simulink model "TEP_Final_NoScript"  (R2024a)
settings: Solver=FixedStepAuto  StartTime=0.0  StopTime=10  FixedStep=1/3600  RelTol=1e-3
model workspace (MAT data in the model file):
  AD : Simulink.Parameter (value not decoded)
  AG : Simulink.Parameter (value not decoded)
  AH : Simulink.Parameter (value not decoded)
  AV : Simulink.Parameter (value not decoded)
  AVP : Simulink.Parameter (value not decoded)
  BCHL : Simulink.Parameter (value not decoded)
  BCHV : Simulink.Parameter (value not decoded)
  BD : Simulink.Parameter (value not decoded)
  BG : Simulink.Parameter (value not decoded)
  BH : Simulink.Parameter (value not decoded)
  BVP : Simulink.Parameter (value not decoded)
  CD : Simulink.Parameter (value not decoded)
  CG : Simulink.Parameter (value not decoded)
  CH : Simulink.Parameter (value not decoded)
  CVP : Simulink.Parameter (value not decoded)
  XMW : Simulink.Parameter (value not decoded)
  XNS : Simulink.Parameter (value not decoded)
  XNSE : Simulink.Parameter (value not decoded)
symbols that are objects in the model workspace (value not decoded): AD, AG, AH, AV, AVP, BD, BG, BH, BVP, CD, CG, CH, CVP, XMW, XNS, XNSE
undefined symbols (not defined in the file or in its folder): magnitude, msgbox, SETPT, XMEAS, XMV
libraries: mylib x360, dspindex x28
(part 11 of 14)

== system TEP_Final_NoScript/Subsystem1/Stripper recycle stream/Composition measurement mol%/Subsystem ==
  XST : Inport
  XMNSE : Inport  Port=2
  Bus Selector : BusSelector  OutputSignals=XMNSEA,XMNSEB,XMNSEC,XMNSED,XMNSEE,XMNSEF,XMNSEG,XMNSEH
  Process Noise I=23-{1..7,36} (8 alike) : mylib/Process Noise I=23-36  SystemSampleTime=-1  VariantActivationTime=update diagram  AllowFlexibleInterface=on  Latency=0  AutoFrameSizeCalculation=off
      settings: SourceProductName=TEP Library
  Subsystem : Subsystem
  SMEASXA : Outport  VectorParamsAs1DForOutWhenUnconnected=off
  SMEASXB : Outport  Port=2  VectorParamsAs1DForOutWhenUnconnected=off
  SMEASXC : Outport  Port=3  VectorParamsAs1DForOutWhenUnconnected=off
  SMEASXD : Outport  Port=4  VectorParamsAs1DForOutWhenUnconnected=off
  SMEASXE : Outport  Port=5  VectorParamsAs1DForOutWhenUnconnected=off
  SMEASXF : Outport  Port=6  VectorParamsAs1DForOutWhenUnconnected=off
  SMEASXG : Outport  Port=7  VectorParamsAs1DForOutWhenUnconnected=off
  SMEASXH : Outport  Port=8  VectorParamsAs1DForOutWhenUnconnected=off
  wires:
  Process Noise I=23-36/1 -> SMEASXA/1
  Process Noise I=23-1/1 -> SMEASXB/1
  Bus Selector/2 -> Process Noise I=23-1/2  "<XMNSEB>"
  Process Noise I=23-2/1 -> SMEASXC/1
  Process Noise I=23-3/1 -> SMEASXD/1
  Process Noise I=23-4/1 -> SMEASXE/1
  Process Noise I=23-5/1 -> SMEASXF/1
  Process Noise I=23-6/1 -> SMEASXG/1
  Process Noise I=23-7/1 -> SMEASXH/1
  Bus Selector/7 -> Process Noise I=23-6/2  "<XMNSEG>"
  Bus Selector/8 -> Process Noise I=23-7/2  "<XMNSEH>"
  Bus Selector/6 -> Process Noise I=23-5/2  "<XMNSEF>"
  Bus Selector/5 -> Process Noise I=23-4/2  "<XMNSEE>"
  Bus Selector/4 -> Process Noise I=23-3/2  "<XMNSED>"
  Bus Selector/3 -> Process Noise I=23-2/2  "<XMNSEC>"
  Bus Selector/1 -> Process Noise I=23-36/2  "<XMNSEA>"
  XST/1 -> Subsystem/1(XST)
  Subsystem/1(XCMPA) -> Process Noise I=23-36/1
  Subsystem/2(XCMPB) -> Process Noise I=23-1/1
  Subsystem/3(XCMPC) -> Process Noise I=23-2/1
  Subsystem/4(XCMPD) -> Process Noise I=23-3/1
  Subsystem/5("XCMPE ") -> Process Noise I=23-4/1
  Subsystem/6("XCMPF ") -> Process Noise I=23-5/1
  Subsystem/7(XCMPG) -> Process Noise I=23-6/1
  Subsystem/8("XCMPH ") -> Process Noise I=23-7/1
  XMNSE/1 -> Bus Selector/1

== system TEP_Final_NoScript/Subsystem1/Stripper recycle stream/Flow measurement in kg//h/XMWS Molecular weight of Stream lb//lb-mol ==
  XST : Inport
  Product : Product
  Sum of Elements : Sum  Inputs=+
  "XMW(I) Molecular weight of components lb/lb-mol " : Constant  Value=XMW
  XMWS : Outport  VectorParamsAs1DForOutWhenUnconnected=off
  wires:
  Sum of Elements/1 -> XMWS/1
  Product/1 -> Sum of Elements/1
  XST/1 -> Product/1
  "XMW(I) Molecular weight of components lb/lb-mol "/1 -> Product/2

== system TEP_Final_NoScript/Subsystem1/Subsystem1/Subsystem1/Composition measurement fraction ==
  X in % : Inport
  Constant : Constant  Value=100
  Divide : Product  Inputs=*/
  SMEASX : Outport
  wires:
  X in %/1 -> Divide/1
  Constant/1 -> Divide/2
  Divide/1 -> SMEASX/1

== system TEP_Final_NoScript/Subsystem1/Subsystem1/Subsystem1/Flow measurement in lb-mol//hr ==
  F in kg/h : Inport
  XST : Inport  Port=2
  Convert from kg/h to lb/h : Constant  Value=2.20462
  Divide : Product  Inputs=**/
  XMWS Molecular weight of Stream lb/lb-mol : Subsystem
  "SMEASF " : Outport  VectorParamsAs1DForOutWhenUnconnected=off
  wires:
  Convert from kg/h to lb/h/1 -> Divide/2
  F in kg/h/1 -> Divide/1
  XMWS Molecular weight of Stream lb/lb-mol/1(XMWS) -> Divide/3
  Divide/1 -> "SMEASF "/1
  XST/1 -> XMWS Molecular weight of Stream lb/lb-mol/1(XST)

== system TEP_Final_NoScript/Subsystem1/Subsystem1/Subsystem1/Pressure measurement in mmHg ==
  "P in kPa " : Inport
  " mm Hg   " : Constant  Value=7.50062
  Pressure conversion mm Hg : Product  Inputs=**
  SMEASP : Outport  VectorParamsAs1DForOutWhenUnconnected=off
  wires:
  "P in kPa "/1 -> Pressure conversion mm Hg/1
  " mm Hg   "/1 -> Pressure conversion mm Hg/2
  Pressure conversion mm Hg/1 -> SMEASP/1

== system TEP_Final_NoScript/Subsystem1/Subsystem13/Subsystem1/Composition measurement fraction ==
  X in % : Inport
  Constant : Constant  Value=100
  Divide : Product  Inputs=*/
  SMEASX : Outport
  wires:
  X in %/1 -> Divide/1
  Constant/1 -> Divide/2
  Divide/1 -> SMEASX/1

== system TEP_Final_NoScript/Subsystem1/Subsystem13/Subsystem1/Flow measurement in lb-mol//hr ==
  F in kg/h : Inport
  XST : Inport  Port=2
  Convert from kg/h to lb/h : Constant  Value=2.20462
  Divide : Product  Inputs=**/
  XMWS Molecular weight of Stream lb/lb-mol : Subsystem
  "SMEASF " : Outport  VectorParamsAs1DForOutWhenUnconnected=off
  wires:
  Convert from kg/h to lb/h/1 -> Divide/2
  F in kg/h/1 -> Divide/1
  XMWS Molecular weight of Stream lb/lb-mol/1(XMWS) -> Divide/3
  Divide/1 -> "SMEASF "/1
  XST/1 -> XMWS Molecular weight of Stream lb/lb-mol/1(XST)

== system TEP_Final_NoScript/Subsystem1/Subsystem13/Subsystem1/Pressure measurement in mmHg ==
  "P in kPa " : Inport
  " mm Hg   " : Constant  Value=7.50062
  Pressure conversion mm Hg : Product  Inputs=**
  SMEASP : Outport  VectorParamsAs1DForOutWhenUnconnected=off
  wires:
  "P in kPa "/1 -> Pressure conversion mm Hg/1
  " mm Hg   "/1 -> Pressure conversion mm Hg/2
  Pressure conversion mm Hg/1 -> SMEASP/1

== system TEP_Final_NoScript/Subsystem1/Subsystem14/Subsystem1/Composition measurement fraction ==
  X in % : Inport
  Constant : Constant  Value=100
  Divide : Product  Inputs=*/
  SMEASX : Outport
  wires:
  X in %/1 -> Divide/1
  Constant/1 -> Divide/2
  Divide/1 -> SMEASX/1

== system TEP_Final_NoScript/Subsystem1/Subsystem14/Subsystem1/Flow measurement in lb-mol//hr ==
  F in kg/h : Inport
  XST : Inport  Port=2
  Convert from kg/h to lb/h : Constant  Value=2.20462
  Divide : Product  Inputs=**/
  XMWS Molecular weight of Stream lb/lb-mol : Subsystem
  "SMEASF " : Outport  VectorParamsAs1DForOutWhenUnconnected=off
  wires:
  Convert from kg/h to lb/h/1 -> Divide/2
  F in kg/h/1 -> Divide/1
  XMWS Molecular weight of Stream lb/lb-mol/1(XMWS) -> Divide/3
  Divide/1 -> "SMEASF "/1
  XST/1 -> XMWS Molecular weight of Stream lb/lb-mol/1(XST)

== system TEP_Final_NoScript/Subsystem1/Subsystem14/Subsystem1/Pressure measurement in mmHg ==
  "P in kPa " : Inport
  " mm Hg   " : Constant  Value=7.50062
  Pressure conversion mm Hg : Product  Inputs=**
  SMEASP : Outport  VectorParamsAs1DForOutWhenUnconnected=off
  wires:
  "P in kPa "/1 -> Pressure conversion mm Hg/1
  " mm Hg   "/1 -> Pressure conversion mm Hg/2
  Pressure conversion mm Hg/1 -> SMEASP/1

== system TEP_Final_NoScript/Subsystem1/Subsystem15/Subsystem1/Composition measurement fraction ==
  X in % : Inport
  Constant : Constant  Value=100
  Divide : Product  Inputs=*/
  SMEASX : Outport
  wires:
  X in %/1 -> Divide/1
  Constant/1 -> Divide/2
  Divide/1 -> SMEASX/1

== system TEP_Final_NoScript/Subsystem1/Subsystem15/Subsystem1/Flow measurement in lb-mol//hr ==
  F in kg/h : Inport
  XST : Inport  Port=2
  Convert from kg/h to lb/h : Constant  Value=2.20462
  Divide : Product  Inputs=**/
  XMWS Molecular weight of Stream lb/lb-mol : Subsystem
  "SMEASF " : Outport  VectorParamsAs1DForOutWhenUnconnected=off
  wires:
  Convert from kg/h to lb/h/1 -> Divide/2
  F in kg/h/1 -> Divide/1
  XMWS Molecular weight of Stream lb/lb-mol/1(XMWS) -> Divide/3
  Divide/1 -> "SMEASF "/1
  XST/1 -> XMWS Molecular weight of Stream lb/lb-mol/1(XST)

== system TEP_Final_NoScript/Subsystem1/Subsystem15/Subsystem1/Pressure measurement in mmHg ==
  "P in kPa " : Inport
  " mm Hg   " : Constant  Value=7.50062
  Pressure conversion mm Hg : Product  Inputs=**
  SMEASP : Outport  VectorParamsAs1DForOutWhenUnconnected=off
  wires:
  "P in kPa "/1 -> Pressure conversion mm Hg/1
  " mm Hg   "/1 -> Pressure conversion mm Hg/2
  Pressure conversion mm Hg/1 -> SMEASP/1

== system TEP_Final_NoScript/Subsystem1/Subsystem16/Subsystem1/Composition measurement fraction ==
  X in % : Inport
  Constant : Constant  Value=100
  Divide : Product  Inputs=*/
  SMEASX : Outport
  wires:
  X in %/1 -> Divide/1
  Constant/1 -> Divide/2
  Divide/1 -> SMEASX/1

== system TEP_Final_NoScript/Subsystem1/Subsystem16/Subsystem1/Flow measurement in lb-mol//hr ==
  F in kg/h : Inport
  XST : Inport  Port=2
  Convert from kg/h to lb/h : Constant  Value=2.20462
  Divide : Product  Inputs=**/
  XMWS Molecular weight of Stream lb/lb-mol : Subsystem
  "SMEASF " : Outport  VectorParamsAs1DForOutWhenUnconnected=off
  wires:
  Convert from kg/h to lb/h/1 -> Divide/2
  F in kg/h/1 -> Divide/1
  XMWS Molecular weight of Stream lb/lb-mol/1(XMWS) -> Divide/3
  Divide/1 -> "SMEASF "/1
  XST/1 -> XMWS Molecular weight of Stream lb/lb-mol/1(XST)

== system TEP_Final_NoScript/Subsystem1/Subsystem16/Subsystem1/Pressure measurement in mmHg ==
  "P in kPa " : Inport
  " mm Hg   " : Constant  Value=7.50062
  Pressure conversion mm Hg : Product  Inputs=**
  SMEASP : Outport  VectorParamsAs1DForOutWhenUnconnected=off
  wires:
  "P in kPa "/1 -> Pressure conversion mm Hg/1
  " mm Hg   "/1 -> Pressure conversion mm Hg/2
  Pressure conversion mm Hg/1 -> SMEASP/1

== system TEP_Final_NoScript/Subsystem1/Subsystem17/Subsystem1/Composition measurement fraction ==
  X in % : Inport
  Constant : Constant  Value=100
  Divide : Product  Inputs=*/
  SMEASX : Outport
  wires:
  X in %/1 -> Divide/1
  Constant/1 -> Divide/2
  Divide/1 -> SMEASX/1

== system TEP_Final_NoScript/Subsystem1/Subsystem17/Subsystem1/Flow measurement in lb-mol//hr ==
  F in kg/h : Inport
  XST : Inport  Port=2
  Convert from kg/h to lb/h : Constant  Value=2.20462
  Divide : Product  Inputs=**/
  XMWS Molecular weight of Stream lb/lb-mol : Subsystem
  "SMEASF " : Outport  VectorParamsAs1DForOutWhenUnconnected=off
  wires:
  Convert from kg/h to lb/h/1 -> Divide/2
  F in kg/h/1 -> Divide/1
  XMWS Molecular weight of Stream lb/lb-mol/1(XMWS) -> Divide/3
  Divide/1 -> "SMEASF "/1
  XST/1 -> XMWS Molecular weight of Stream lb/lb-mol/1(XST)

== system TEP_Final_NoScript/Subsystem1/Subsystem17/Subsystem1/Pressure measurement in mmHg ==
  "P in kPa " : Inport
  " mm Hg   " : Constant  Value=7.50062
  Pressure conversion mm Hg : Product  Inputs=**
  SMEASP : Outport  VectorParamsAs1DForOutWhenUnconnected=off
  wires:
  "P in kPa "/1 -> Pressure conversion mm Hg/1
  " mm Hg   "/1 -> Pressure conversion mm Hg/2
  Pressure conversion mm Hg/1 -> SMEASP/1

== system TEP_Final_NoScript/Subsystem1/Subsystem2/Subsystem1/Composition measurement fraction ==
  X in % : Inport
  Constant : Constant  Value=100
  Divide : Product  Inputs=*/
  SMEASX : Outport
  wires:
  X in %/1 -> Divide/1
  Constant/1 -> Divide/2
  Divide/1 -> SMEASX/1

== system TEP_Final_NoScript/Subsystem1/Subsystem2/Subsystem1/Flow measurement in lb-mol//hr ==
  F in kg/h : Inport
  XST : Inport  Port=2
  Convert from kg/h to lb/h : Constant  Value=2.20462
  Divide : Product  Inputs=**/
  XMWS Molecular weight of Stream lb/lb-mol : Subsystem
  "SMEASF " : Outport  VectorParamsAs1DForOutWhenUnconnected=off
  wires:
  Convert from kg/h to lb/h/1 -> Divide/2
  F in kg/h/1 -> Divide/1
  XMWS Molecular weight of Stream lb/lb-mol/1(XMWS) -> Divide/3
  Divide/1 -> "SMEASF "/1
  XST/1 -> XMWS Molecular weight of Stream lb/lb-mol/1(XST)

== system TEP_Final_NoScript/Subsystem1/Subsystem2/Subsystem1/Pressure measurement in mmHg ==
  "P in kPa " : Inport
  " mm Hg   " : Constant  Value=7.50062
  Pressure conversion mm Hg : Product  Inputs=**
  SMEASP : Outport  VectorParamsAs1DForOutWhenUnconnected=off
  wires:
  "P in kPa "/1 -> Pressure conversion mm Hg/1
  " mm Hg   "/1 -> Pressure conversion mm Hg/2
  Pressure conversion mm Hg/1 -> SMEASP/1

== system TEP_Final_NoScript/Subsystem1/Subsystem3/Subsystem1/Composition measurement fraction ==
  X in % : Inport
  Constant : Constant  Value=100
  Divide : Product  Inputs=*/
  SMEASX : Outport
  wires:
  X in %/1 -> Divide/1
  Constant/1 -> Divide/2
  Divide/1 -> SMEASX/1

== system TEP_Final_NoScript/Subsystem1/Subsystem3/Subsystem1/Flow measurement in lb-mol//hr ==
  F in kg/h : Inport
  XST : Inport  Port=2
  Convert from kg/h to lb/h : Constant  Value=2.20462
  Divide : Product  Inputs=**/
  XMWS Molecular weight of Stream lb/lb-mol : Subsystem
  "SMEASF " : Outport  VectorParamsAs1DForOutWhenUnconnected=off
  wires:
  Convert from kg/h to lb/h/1 -> Divide/2
  F in kg/h/1 -> Divide/1
  XMWS Molecular weight of Stream lb/lb-mol/1(XMWS) -> Divide/3
  Divide/1 -> "SMEASF "/1
  XST/1 -> XMWS Molecular weight of Stream lb/lb-mol/1(XST)

== system TEP_Final_NoScript/Subsystem1/Subsystem3/Subsystem1/Pressure measurement in mmHg ==
  "P in kPa " : Inport
  " mm Hg   " : Constant  Value=7.50062
  Pressure conversion mm Hg : Product  Inputs=**
  SMEASP : Outport  VectorParamsAs1DForOutWhenUnconnected=off
  wires:
  "P in kPa "/1 -> Pressure conversion mm Hg/1
  " mm Hg   "/1 -> Pressure conversion mm Hg/2
  Pressure conversion mm Hg/1 -> SMEASP/1

== system TEP_Final_NoScript/Subsystem1/Subsystem4/Subsystem1/Composition measurement fraction ==
  X in % : Inport
  Constant : Constant  Value=100
  Divide : Product  Inputs=*/
  SMEASX : Outport
  wires:
  X in %/1 -> Divide/1
  Constant/1 -> Divide/2
  Divide/1 -> SMEASX/1

== system TEP_Final_NoScript/Subsystem1/Subsystem4/Subsystem1/Flow measurement in lb-mol//hr ==
  F in kg/h : Inport
  XST : Inport  Port=2
  Convert from kg/h to lb/h : Constant  Value=2.20462
  Divide : Product  Inputs=**/
  XMWS Molecular weight of Stream lb/lb-mol : Subsystem
  "SMEASF " : Outport  VectorParamsAs1DForOutWhenUnconnected=off
  wires:
  Convert from kg/h to lb/h/1 -> Divide/2
  F in kg/h/1 -> Divide/1
  XMWS Molecular weight of Stream lb/lb-mol/1(XMWS) -> Divide/3
  Divide/1 -> "SMEASF "/1
  XST/1 -> XMWS Molecular weight of Stream lb/lb-mol/1(XST)

== system TEP_Final_NoScript/Subsystem1/Subsystem4/Subsystem1/Pressure measurement in mmHg ==
  "P in kPa " : Inport
  " mm Hg   " : Constant  Value=7.50062
  Pressure conversion mm Hg : Product  Inputs=**
  SMEASP : Outport  VectorParamsAs1DForOutWhenUnconnected=off
  wires:
  "P in kPa "/1 -> Pressure conversion mm Hg/1
  " mm Hg   "/1 -> Pressure conversion mm Hg/2
  Pressure conversion mm Hg/1 -> SMEASP/1

== system TEP_Final_NoScript/Subsystem1/Subsystem5/Subsystem1/Composition measurement fraction ==
  X in % : Inport
  Constant : Constant  Value=100
  Divide : Product  Inputs=*/
  SMEASX : Outport
  wires:
  X in %/1 -> Divide/1
  Constant/1 -> Divide/2
  Divide/1 -> SMEASX/1

== system TEP_Final_NoScript/Subsystem1/Subsystem5/Subsystem1/Flow measurement in lb-mol//hr ==
  F in kg/h : Inport
  XST : Inport  Port=2
  Convert from kg/h to lb/h : Constant  Value=2.20462
  Divide : Product  Inputs=**/
  XMWS Molecular weight of Stream lb/lb-mol : Subsystem
  "SMEASF " : Outport  VectorParamsAs1DForOutWhenUnconnected=off
  wires:
  Convert from kg/h to lb/h/1 -> Divide/2
  F in kg/h/1 -> Divide/1
  XMWS Molecular weight of Stream lb/lb-mol/1(XMWS) -> Divide/3
  Divide/1 -> "SMEASF "/1
  XST/1 -> XMWS Molecular weight of Stream lb/lb-mol/1(XST)

== system TEP_Final_NoScript/Subsystem1/Subsystem5/Subsystem1/Pressure measurement in mmHg ==
  "P in kPa " : Inport
  " mm Hg   " : Constant  Value=7.50062
  Pressure conversion mm Hg : Product  Inputs=**
  SMEASP : Outport  VectorParamsAs1DForOutWhenUnconnected=off
  wires:
  "P in kPa "/1 -> Pressure conversion mm Hg/1
  " mm Hg   "/1 -> Pressure conversion mm Hg/2
  Pressure conversion mm Hg/1 -> SMEASP/1

== system TEP_Final_NoScript/Subsystem1/Subsystem8/Subsystem1/Composition measurement fraction ==
  X in % : Inport
  Constant : Constant  Value=100
  Divide : Product  Inputs=*/
  SMEASX : Outport
  wires:
  X in %/1 -> Divide/1
  Constant/1 -> Divide/2
  Divide/1 -> SMEASX/1

== system TEP_Final_NoScript/Subsystem1/Subsystem8/Subsystem1/Flow measurement in lb-mol//hr ==
  F in kg/h : Inport
  XST : Inport  Port=2
  Convert from kg/h to lb/h : Constant  Value=2.20462
  Divide : Product  Inputs=**/
  XMWS Molecular weight of Stream lb/lb-mol : Subsystem
  "SMEASF " : Outport  VectorParamsAs1DForOutWhenUnconnected=off
  wires:
  Convert from kg/h to lb/h/1 -> Divide/2
  F in kg/h/1 -> Divide/1
  XMWS Molecular weight of Stream lb/lb-mol/1(XMWS) -> Divide/3
  Divide/1 -> "SMEASF "/1
  XST/1 -> XMWS Molecular weight of Stream lb/lb-mol/1(XST)

== system TEP_Final_NoScript/Subsystem1/Subsystem8/Subsystem1/Pressure measurement in mmHg ==
  "P in kPa " : Inport
  " mm Hg   " : Constant  Value=7.50062
  Pressure conversion mm Hg : Product  Inputs=**
  SMEASP : Outport  VectorParamsAs1DForOutWhenUnconnected=off
  wires:
  "P in kPa "/1 -> Pressure conversion mm Hg/1
  " mm Hg   "/1 -> Pressure conversion mm Hg/2
  Pressure conversion mm Hg/1 -> SMEASP/1

== system TEP_Final_NoScript/Random number generator1/Process Measurements XMEAS(I) I=23-36/Gas Analysis Delay/Subsystem/If Action Subsystem ==
  Action Port : ActionPort  ActionPortLabel=if(u1 == u2)
  Constant : Constant  Value=0
  Out1 : Outport  VectorParamsAs1DForOutWhenUnconnected=off
  wires:
  Constant/1 -> Out1/1

== system TEP_Final_NoScript/Random number generator1/Process Measurements XMEAS(I) I=23-36/Gas Analysis Delay/Subsystem/If Action Subsystem1 ==
  In1 : Inport
  Action Port : ActionPort  ActionPortLabel=else
  Out1 : Outport  VectorParamsAs1DForOutWhenUnconnected=off
  wires:
  In1/1 -> Out1/1

== system TEP_Final_NoScript/Random number generator1/Process Measurements XMEAS(I) I=23-36/If Action Subsystem3/Subsystem/Subsystem ==
  G : Inport
  TESUB6 XMNS(23) : Subsystem
  TESUB6 XMNS(24) : Subsystem
  TESUB6 XMNS(25) : Subsystem
  TESUB6 XMNS(26) : Subsystem
  TESUB6 XMNS(27) : Subsystem
  XMNS(23) : Outport  VectorParamsAs1DForOutWhenUnconnected=off
  XMNS(24) : Outport  Port=2  VectorParamsAs1DForOutWhenUnconnected=off
  XMNS(25) : Outport  Port=3  VectorParamsAs1DForOutWhenUnconnected=off
  XMNS(26) : Outport  Port=4  VectorParamsAs1DForOutWhenUnconnected=off
  XMNS(27) : Outport  Port=5  VectorParamsAs1DForOutWhenUnconnected=off
  G_NEW : Outport  Port=6  VectorParamsAs1DForOutWhenUnconnected=off
  wires:
  TESUB6 XMNS(24)/2(G_NEW) -> TESUB6 XMNS(25)/1(G)
  G/1 -> TESUB6 XMNS(23)/1(G)
  TESUB6 XMNS(23)/2(G_NEW) -> TESUB6 XMNS(24)/1(G)
  TESUB6 XMNS(25)/2(G_NEW) -> TESUB6 XMNS(26)/1(G)
  TESUB6 XMNS(26)/1(XMNS) -> XMNS(26)/1  "XMNS(26)"
  TESUB6 XMNS(27)/1(XMNS) -> XMNS(27)/1  "XMNS(27)"
  TESUB6 XMNS(27)/2(G_NEW) -> G_NEW/1
  TESUB6 XMNS(26)/2(G_NEW) -> TESUB6 XMNS(27)/1(G)
  TESUB6 XMNS(25)/1(XMNS) -> XMNS(25)/1  "XMNS(25)"
  TESUB6 XMNS(23)/1(XMNS) -> XMNS(23)/1  "XMNS(23)"
  TESUB6 XMNS(24)/1(XMNS) -> XMNS(24)/1  "XMNS(24)"

== system TEP_Final_NoScript/Random number generator1/Process Measurements XMEAS(I) I=23-36/If Action Subsystem3/Subsystem/Subsystem1 ==
  G : Inport
  TESUB6 XMNS(28) : Subsystem
  TESUB6 XMNS(29) : Subsystem
  TESUB6 XMNS(30) : Subsystem
  TESUB6 XMNS(31) : Subsystem
  TESUB6 XMNS(32) : Subsystem
  XMNS(28) : Outport  VectorParamsAs1DForOutWhenUnconnected=off
  XMNS(29) : Outport  Port=2  VectorParamsAs1DForOutWhenUnconnected=off
  XMNS(30) : Outport  Port=3  VectorParamsAs1DForOutWhenUnconnected=off
  XMNS(31) : Outport  Port=4  VectorParamsAs1DForOutWhenUnconnected=off
  XMNS(32) : Outport  Port=5  VectorParamsAs1DForOutWhenUnconnected=off
  G_NEW : Outport  Port=6  VectorParamsAs1DForOutWhenUnconnected=off
  wires:
  TESUB6 XMNS(29)/2(G_NEW) -> TESUB6 XMNS(30)/1(G)
  G/1 -> TESUB6 XMNS(28)/1(G)
  TESUB6 XMNS(28)/2(G_NEW) -> TESUB6 XMNS(29)/1(G)
  TESUB6 XMNS(30)/2(G_NEW) -> TESUB6 XMNS(31)/1(G)
  TESUB6 XMNS(31)/1(XMNS) -> XMNS(31)/1  "XMNS(31)"
  TESUB6 XMNS(32)/1(XMNS) -> XMNS(32)/1  "XMNS(32)"
  TESUB6 XMNS(32)/2(G_NEW) -> G_NEW/1
  TESUB6 XMNS(31)/2(G_NEW) -> TESUB6 XMNS(32)/1(G)
  TESUB6 XMNS(30)/1(XMNS) -> XMNS(30)/1  "XMNS(30)"
  TESUB6 XMNS(28)/1(XMNS) -> XMNS(28)/1  "XMNS(28)"
  TESUB6 XMNS(29)/1(XMNS) -> XMNS(29)/1  "XMNS(29)"

== system TEP_Final_NoScript/Random number generator1/Process Measurements XMEAS(I) I=23-36/If Action Subsystem3/Subsystem/Subsystem2 ==
  G : Inport
  TESUB6 XMNS(33) : Subsystem
  TESUB6 XMNS(34) : Subsystem
  TESUB6 XMNS(35) : Subsystem
  TESUB6 XMNS(36) : Subsystem
  XMNS(33) : Outport  VectorParamsAs1DForOutWhenUnconnected=off
  XMNS(34) : Outport  Port=2  VectorParamsAs1DForOutWhenUnconnected=off
  XMNS(35) : Outport  Port=3  VectorParamsAs1DForOutWhenUnconnected=off
  XMNS(36) : Outport  Port=4  VectorParamsAs1DForOutWhenUnconnected=off
  G_NEW : Outport  Port=5  VectorParamsAs1DForOutWhenUnconnected=off
  wires:
  TESUB6 XMNS(34)/2(G_NEW) -> TESUB6 XMNS(35)/1(G)
  G/1 -> TESUB6 XMNS(33)/1(G)
  TESUB6 XMNS(33)/2(G_NEW) -> TESUB6 XMNS(34)/1(G)
  TESUB6 XMNS(35)/2(G_NEW) -> TESUB6 XMNS(36)/1(G)
  TESUB6 XMNS(36)/1(XMNS) -> XMNS(36)/1  "XMNS(36)"
  TESUB6 XMNS(36)/2(G_NEW) -> G_NEW/1
  TESUB6 XMNS(35)/1(XMNS) -> XMNS(35)/1  "XMNS(35)"
  TESUB6 XMNS(33)/1(XMNS) -> XMNS(33)/1  "XMNS(33)"
  TESUB6 XMNS(34)/1(XMNS) -> XMNS(34)/1  "XMNS(34)"

== system TEP_Final_NoScript/Random number generator1/Process Measurements XMEAS(I) I=37-41/Gas Analysis Delay/Subsystem/If Action Subsystem ==
  Action Port : ActionPort  ActionPortLabel=if(u1 == u2)
  Constant : Constant  Value=0
  Out1 : Outport  VectorParamsAs1DForOutWhenUnconnected=off
  wires:
  Constant/1 -> Out1/1

== system TEP_Final_NoScript/Random number generator1/Process Measurements XMEAS(I) I=37-41/Gas Analysis Delay/Subsystem/If Action Subsystem1 ==
  In1 : Inport
  Action Port : ActionPort  ActionPortLabel=else
  Out1 : Outport  VectorParamsAs1DForOutWhenUnconnected=off
  wires:
  In1/1 -> Out1/1

== system TEP_Final_NoScript/Random number generator1/Process Measurements XMEAS(I) I=37-41/If Action Subsystem3/Subsystem/Subsystem ==
  G : Inport
  TESUB6 XMNS(37) : Subsystem
  TESUB6 XMNS(38) : Subsystem
  TESUB6 XMNS(39) : Subsystem
  TESUB6 XMNS(40) : Subsystem
  TESUB6 XMNS(41) : Subsystem
  XMNS(37) : Outport  VectorParamsAs1DForOutWhenUnconnected=off
  XMNS(38) : Outport  Port=2  VectorParamsAs1DForOutWhenUnconnected=off
  XMNS(39) : Outport  Port=3  VectorParamsAs1DForOutWhenUnconnected=off
  XMNS(40) : Outport  Port=4  VectorParamsAs1DForOutWhenUnconnected=off
  XMNS(41) : Outport  Port=5  VectorParamsAs1DForOutWhenUnconnected=off
  G_NEW : Outport  Port=6  VectorParamsAs1DForOutWhenUnconnected=off
  wires:
  TESUB6 XMNS(38)/2(G_NEW) -> TESUB6 XMNS(39)/1(G)
  G/1 -> TESUB6 XMNS(37)/1(G)
  TESUB6 XMNS(37)/2(G_NEW) -> TESUB6 XMNS(38)/1(G)
  TESUB6 XMNS(39)/2(G_NEW) -> TESUB6 XMNS(40)/1(G)
  TESUB6 XMNS(40)/1(XMNS) -> XMNS(40)/1  "XMNS(40)"
  TESUB6 XMNS(41)/1(XMNS) -> XMNS(41)/1  "XMNS(41)"
  TESUB6 XMNS(41)/2(G_NEW) -> G_NEW/1
  TESUB6 XMNS(40)/2(G_NEW) -> TESUB6 XMNS(41)/1(G)
  TESUB6 XMNS(39)/1(XMNS) -> XMNS(39)/1  "XMNS(39)"
  TESUB6 XMNS(37)/1(XMNS) -> XMNS(37)/1  "XMNS(37)"
  TESUB6 XMNS(38)/1(XMNS) -> XMNS(38)/1  "XMNS(38)"

== system TEP_Final_NoScript/Random number generator1/Stream Measurements SMEAS Gas analysis/Gas Analysis Delay/Subsystem/If Action Subsystem ==
  Action Port : ActionPort  ActionPortLabel=if(u1 == u2)
  Constant : Constant  Value=0
  Out1 : Outport  VectorParamsAs1DForOutWhenUnconnected=off
  wires:
  Constant/1 -> Out1/1

== system TEP_Final_NoScript/Random number generator1/Stream Measurements SMEAS Gas analysis/Gas Analysis Delay/Subsystem/If Action Subsystem1 ==
  In1 : Inport
  Action Port : ActionPort  ActionPortLabel=else
  Out1 : Outport  VectorParamsAs1DForOutWhenUnconnected=off
  wires:
  In1/1 -> Out1/1

== system TEP_Final_NoScript/Random number generator1/Stream Measurements SMEAS Gas analysis/If Action Subsystem3/Subsystem/Stream 1 ==
  G : Inport
  Bus Creator : BusCreator  Inputs=8
  Subsystem : Subsystem
  Stream 1 : Outport
  G_NEW : Outport  Port=2
  wires:
  Subsystem/4(XMNSED) -> Bus Creator/4
  Subsystem/1(XMNSEA) -> Bus Creator/1
  G/1 -> Subsystem/1(G)
  Subsystem/8(XMNSEH) -> Bus Creator/8
  Subsystem/3(XMNSEC) -> Bus Creator/3
  Subsystem/7(XMNSEG) -> Bus Creator/7
  Subsystem/9(G_NEW) -> G_NEW/1
  Subsystem/2(XMNSEB) -> Bus Creator/2
  Subsystem/5(XMNSEE) -> Bus Creator/5
  Subsystem/6(XMNSEF) -> Bus Creator/6
  Bus Creator/1 -> Stream 1/1  "Stream 1"

== system TEP_Final_NoScript/Random number generator1/Stream Measurements SMEAS Gas analysis/If Action Subsystem3/Subsystem/Stream 13 ==
  G : Inport
  Bus Creator : BusCreator  Inputs=8
  Subsystem : Subsystem
  Stream 13 : Outport
  G_NEW : Outport  Port=2
  wires:
  Subsystem/4(XMNSED) -> Bus Creator/4
  Subsystem/1(XMNSEA) -> Bus Creator/1
  G/1 -> Subsystem/1(G)
  Subsystem/8(XMNSEH) -> Bus Creator/8
  Subsystem/3(XMNSEC) -> Bus Creator/3
  Subsystem/7(XMNSEG) -> Bus Creator/7
  Subsystem/9(G_NEW) -> G_NEW/1
  Subsystem/2(XMNSEB) -> Bus Creator/2
  Subsystem/5(XMNSEE) -> Bus Creator/5
  Subsystem/6(XMNSEF) -> Bus Creator/6
  Bus Creator/1 -> Stream 13/1  "Stream 13"

== system TEP_Final_NoScript/Random number generator1/Stream Measurements SMEAS Gas analysis/If Action Subsystem3/Subsystem/Stream 2 ==
  G : Inport
  Bus Creator : BusCreator  Inputs=8
  Subsystem : Subsystem
  Stream 2 : Outport
  G_NEW : Outport  Port=2
  wires:
  Subsystem/4(XMNSED) -> Bus Creator/4
  Subsystem/1(XMNSEA) -> Bus Creator/1
  G/1 -> Subsystem/1(G)
  Subsystem/8(XMNSEH) -> Bus Creator/8
  Subsystem/3(XMNSEC) -> Bus Creator/3
  Subsystem/7(XMNSEG) -> Bus Creator/7
  Subsystem/9(G_NEW) -> G_NEW/1
  Subsystem/2(XMNSEB) -> Bus Creator/2
  Subsystem/5(XMNSEE) -> Bus Creator/5
  Subsystem/6(XMNSEF) -> Bus Creator/6
  Bus Creator/1 -> Stream 2/1  "Stream 2"

== system TEP_Final_NoScript/Random number generator1/Stream Measurements SMEAS Gas analysis/If Action Subsystem3/Subsystem/Stream 3 ==
  G : Inport
  Bus Creator : BusCreator  Inputs=8
  Subsystem : Subsystem
  Stream 3 : Outport
  G_NEW : Outport  Port=2
  wires:
  Subsystem/4(XMNSED) -> Bus Creator/4
  Subsystem/1(XMNSEA) -> Bus Creator/1
  G/1 -> Subsystem/1(G)
  Subsystem/8(XMNSEH) -> Bus Creator/8
  Subsystem/3(XMNSEC) -> Bus Creator/3
  Subsystem/7(XMNSEG) -> Bus Creator/7
  Subsystem/9(G_NEW) -> G_NEW/1
  Subsystem/2(XMNSEB) -> Bus Creator/2
  Subsystem/5(XMNSEE) -> Bus Creator/5
  Subsystem/6(XMNSEF) -> Bus Creator/6
  Bus Creator/1 -> Stream 3/1  "Stream 3"

== system TEP_Final_NoScript/Random number generator1/Stream Measurements SMEAS Gas analysis/If Action Subsystem3/Subsystem/Stream 4 ==
  G : Inport
  Bus Creator : BusCreator  Inputs=8
  Subsystem : Subsystem
  Stream 4 : Outport
  G_NEW : Outport  Port=2
  wires:
  Subsystem/4(XMNSED) -> Bus Creator/4
  Subsystem/1(XMNSEA) -> Bus Creator/1
  G/1 -> Subsystem/1(G)
  Subsystem/8(XMNSEH) -> Bus Creator/8
  Subsystem/3(XMNSEC) -> Bus Creator/3
  Subsystem/7(XMNSEG) -> Bus Creator/7
  Subsystem/9(G_NEW) -> G_NEW/1
  Subsystem/2(XMNSEB) -> Bus Creator/2
  Subsystem/5(XMNSEE) -> Bus Creator/5
  Subsystem/6(XMNSEF) -> Bus Creator/6
  Bus Creator/1 -> Stream 4/1  "Stream 4"

== system TEP_Final_NoScript/Random number generator1/Stream Measurements SMEAS Gas analysis/If Action Subsystem3/Subsystem/Stream 5 ==
  G : Inport
  Bus Creator : BusCreator  Inputs=8
  Subsystem : Subsystem
  Stream 5 : Outport
  G_NEW : Outport  Port=2
  wires:
  Subsystem/4(XMNSED) -> Bus Creator/4
  Subsystem/1(XMNSEA) -> Bus Creator/1
  G/1 -> Subsystem/1(G)
  Subsystem/8(XMNSEH) -> Bus Creator/8
  Subsystem/3(XMNSEC) -> Bus Creator/3
  Subsystem/7(XMNSEG) -> Bus Creator/7
  Subsystem/9(G_NEW) -> G_NEW/1
  Subsystem/2(XMNSEB) -> Bus Creator/2
  Subsystem/5(XMNSEE) -> Bus Creator/5
  Subsystem/6(XMNSEF) -> Bus Creator/6
  Bus Creator/1 -> Stream 5/1  "Stream 5"

== system TEP_Final_NoScript/Random number generator1/Stream Measurements SMEAS Gas analysis/If Action Subsystem3/Subsystem/Stream 6 ==
  G : Inport
  Bus Creator : BusCreator  Inputs=8
  Subsystem : Subsystem
  Stream 6 : Outport
  G_NEW : Outport  Port=2
  wires:
  Subsystem/4(XMNSED) -> Bus Creator/4
  Subsystem/1(XMNSEA) -> Bus Creator/1
  G/1 -> Subsystem/1(G)
  Subsystem/8(XMNSEH) -> Bus Creator/8
  Subsystem/3(XMNSEC) -> Bus Creator/3
  Subsystem/7(XMNSEG) -> Bus Creator/7
  Subsystem/9(G_NEW) -> G_NEW/1
  Subsystem/2(XMNSEB) -> Bus Creator/2
  Subsystem/5(XMNSEE) -> Bus Creator/5
  Subsystem/6(XMNSEF) -> Bus Creator/6
  Bus Creator/1 -> Stream 6/1  "Stream 6"

== system TEP_Final_NoScript/Random number generator1/Stream Measurements SMEAS Gas analysis/If Action Subsystem3/Subsystem/Stream 8 ==
  G : Inport
  Bus Creator : BusCreator  Inputs=8
  Subsystem : Subsystem
  Stream 8 : Outport
  G_NEW : Outport  Port=2
  wires:
  Subsystem/4(XMNSED) -> Bus Creator/4
  Subsystem/1(XMNSEA) -> Bus Creator/1
  G/1 -> Subsystem/1(G)
  Subsystem/8(XMNSEH) -> Bus Creator/8
  Subsystem/3(XMNSEC) -> Bus Creator/3
  Subsystem/7(XMNSEG) -> Bus Creator/7
  Subsystem/9(G_NEW) -> G_NEW/1
  Subsystem/2(XMNSEB) -> Bus Creator/2
  Subsystem/5(XMNSEE) -> Bus Creator/5
  Subsystem/6(XMNSEF) -> Bus Creator/6
  Bus Creator/1 -> Stream 8/1  "Stream 8"

== system TEP_Final_NoScript/Random number generator1/Stream Measurements SMEAS Gas analysis/If Action Subsystem3/Subsystem/Stream 9 ==
  G : Inport
  Bus Creator : BusCreator  Inputs=8
  Subsystem : Subsystem
  Stream 9 : Outport
  G_NEW : Outport  Port=2
  wires:
  Subsystem/4(XMNSED) -> Bus Creator/4
  Subsystem/1(XMNSEA) -> Bus Creator/1
  G/1 -> Subsystem/1(G)
  Subsystem/8(XMNSEH) -> Bus Creator/8
  Subsystem/3(XMNSEC) -> Bus Creator/3
  Subsystem/7(XMNSEG) -> Bus Creator/7
  Subsystem/9(G_NEW) -> G_NEW/1
  Subsystem/2(XMNSEB) -> Bus Creator/2
  Subsystem/5(XMNSEE) -> Bus Creator/5
  Subsystem/6(XMNSEF) -> Bus Creator/6
  Bus Creator/1 -> Stream 9/1  "Stream 9"

== system TEP_Final_NoScript/Random number generator1/Stream Measurements SMEAS Product analysis/Gas Analysis Delay/Subsystem/If Action Subsystem ==
  Action Port : ActionPort  ActionPortLabel=if(u1 == u2)
  Constant : Constant  Value=0
  Out1 : Outport  VectorParamsAs1DForOutWhenUnconnected=off
  wires:
  Constant/1 -> Out1/1

== system TEP_Final_NoScript/Random number generator1/Stream Measurements SMEAS Product analysis/Gas Analysis Delay/Subsystem/If Action Subsystem1 ==
  In1 : Inport
  Action Port : ActionPort  ActionPortLabel=else
  Out1 : Outport  VectorParamsAs1DForOutWhenUnconnected=off
  wires:
  In1/1 -> Out1/1

== system TEP_Final_NoScript/Random number generator1/Stream Measurements SMEAS Product analysis/If Action Subsystem3/Subsystem/Subsystem1 ==
  G : Inport
  Bus Creator : BusCreator  Inputs=5
  Subsystem : Subsystem
  Stream 11 : Outport
  G_NEW : Outport  Port=2
  wires:
  Subsystem/2(XMNSEE) -> Bus Creator/2
  G/1 -> Subsystem/1(G)
  Subsystem/6(G_NEW) -> G_NEW/1
  Subsystem/5(XMNSEH) -> Bus Creator/5
  Subsystem/4(XMNSEG) -> Bus Creator/4
  Subsystem/3(XMNSEF) -> Bus Creator/3
  Subsystem/1(XMNSED) -> Bus Creator/1
  Bus Creator/1 -> Stream 11/1  "Stream 11"

== system TEP_Final_NoScript/Random number generator1/Stream Measurements SMEAS Product analysis/If Action Subsystem3/Subsystem/Subsystem2 ==
  G : Inport
  Bus Creator : BusCreator  Inputs=5
  Subsystem : Subsystem
  Stream 13 : Outport
  G_NEW : Outport  Port=2
  wires:
  Subsystem/2(XMNSEE) -> Bus Creator/2
  G/1 -> Subsystem/1(G)
  Subsystem/6(G_NEW) -> G_NEW/1
  Subsystem/5(XMNSEH) -> Bus Creator/5
  Subsystem/4(XMNSEG) -> Bus Creator/4
  Subsystem/3(XMNSEF) -> Bus Creator/3
  Subsystem/1(XMNSED) -> Bus Creator/1
  Bus Creator/1 -> Stream 13/1  "Stream 13"

== system TEP_Final_NoScript/Reactor/Reaction Rates/Reaction rates lb-mol//h/Reaction rate of reaction 1 lb-mol//ft3·h/If Action Subsystem ==
  In1 : Inport
  Action Port : ActionPort  ActionPortLabel=if( u1>0 & u2>0 )
  Out1 : Outport  VectorParamsAs1DForOutWhenUnconnected=off
  wires:
  In1/1 -> Out1/1

== system TEP_Final_NoScript/Reactor/Reaction Rates/Reaction rates lb-mol//h/Reaction rate of reaction 1 lb-mol//ft3·h/If Action Subsystem2 ==
  In1 : Inport
  Action Port : ActionPort  ActionPortLabel=else
  Out1 : Outport  VectorParamsAs1DForOutWhenUnconnected=off
  wires:
  In1/1 -> Out1/1

== system TEP_Final_NoScript/Reactor/Reaction Rates/Reaction rates lb-mol//h/Reaction rate of reaction 1 lb-mol//ft3·h/RR(1) Reaction rate of 1st reaction lb-mol//ft3·h  ==
  PPR : Inport
  TKR : Inport  Port=2
  "   " : Constant  Value=1.1544
  "    " : Constant  Value=0.3735
  Abs : Abs  SaturateOnIntegerOverflow=off
  Abs1 : Abs  SaturateOnIntegerOverflow=off
  Activation energy cal/mol : Constant  Value=40000
  Bus Selector : BusSelector  OutputSignals=PPR(1),PPR(3),PPR(4)
  Bus Selector1 : BusSelector  OutputSignals=signal1.TESUB8(7)
  Divide : Product  Inputs=*//
  Divide1 : Product  Inputs=4
  Math Function1 : Math  SignedPower=on
  Preexponential factor lb-mol/ft3·h·mmHg : Constant  Value=31.5859536
  Product : Product
  R1F : Math  Operator=pow  SignedPower=on
  R2F : Math  Operator=pow  SignedPower=on
  Subtract : Sum  Inputs=+-
  Universal gas constant cal/mol·K : Constant  Value=1.987
  RR(1) : Outport  VectorParamsAs1DForOutWhenUnconnected=off
  wires:
  "    "/1 -> R2F/2
  Divide/1 -> Subtract/2
  Universal gas constant cal/mol·K/1 -> Divide/2
  "   "/1 -> R1F/2
  Preexponential factor lb-mol/ft3·h·mmHg/1 -> Subtract/1
  Activation energy cal/mol/1 -> Divide/1
  TKR/1 -> Divide/3
  Subtract/1 -> Math Function1/1
  Divide1/1 -> RR(1)/1
  Bus Selector/2 -> Abs1/1  "<PPR(3)>"
  Abs/1 -> R1F/1
  Abs1/1 -> R2F/1
  PPR/1 -> Bus Selector/1
  Bus Selector/1 -> Abs/1  "<PPR(1)>"
  R1F/1 -> Divide1/2
  R2F/1 -> Divide1/3
  Bus Selector/3 -> Divide1/4  "<PPR(4)>"
  [TESUB8] -> Bus Selector1/1
  Math Function1/1 -> Product/1
  Bus Selector1/1 -> Product/2  "<TESUB8(7)>"
  Product/1 -> Divide1/1

== system TEP_Final_NoScript/Reactor/Reaction Rates/Reaction rates lb-mol//h/Reaction rate of reaction 2 lb-mol//ft3·h/If Action Subsystem ==
  In1 : Inport
  Action Port : ActionPort  ActionPortLabel=if( u1>0 & u2>0)
  Out1 : Outport  VectorParamsAs1DForOutWhenUnconnected=off
  wires:
  In1/1 -> Out1/1

== system TEP_Final_NoScript/Reactor/Reaction Rates/Reaction rates lb-mol//h/Reaction rate of reaction 2 lb-mol//ft3·h/If Action Subsystem2 ==
  In1 : Inport
  Action Port : ActionPort  ActionPortLabel=else
  Out1 : Outport  VectorParamsAs1DForOutWhenUnconnected=off
  wires:
  In1/1 -> Out1/1

== system TEP_Final_NoScript/Reactor/Reaction Rates/Reaction rates lb-mol//h/Reaction rate of reaction 2 lb-mol//ft3·h/RR(2) Reaction rate of 2nd reaction lb-mol//ft3·h  ==
  PPR : Inport
  TKR : Inport  Port=2
  "   " : Constant  Value=1.1544
  "    " : Constant  Value=0.3735
  Abs : Abs  SaturateOnIntegerOverflow=off
  Abs1 : Abs  SaturateOnIntegerOverflow=off
  Activation energy cal/mol : Constant  Value=20000
  Bus Selector : BusSelector  OutputSignals=PPR(1),PPR(3),PPR(5)
  Bus Selector1 : BusSelector  OutputSignals=signal1.TESUB8(8)
  Divide : Product  Inputs=*//
  Divide1 : Product  Inputs=4
  Math Function2 : Math  SignedPower=on
  Preexponential factor lb-mol/ft3·h·mmHg : Constant  Value=3.00094014
  Product : Product
  R1F : Math  Operator=pow  SignedPower=on
  R2F : Math  Operator=pow  SignedPower=on
  Subtract : Sum  Inputs=+-
  Universal gas constant cal/mol·K : Constant  Value=1.987
  RR(2) : Outport  VectorParamsAs1DForOutWhenUnconnected=off
  wires:
  "    "/1 -> R2F/2
  Divide/1 -> Subtract/2
  Universal gas constant cal/mol·K/1 -> Divide/2
  "   "/1 -> R1F/2
  Preexponential factor lb-mol/ft3·h·mmHg/1 -> Subtract/1
  Activation energy cal/mol/1 -> Divide/1
  TKR/1 -> Divide/3
  Subtract/1 -> Math Function2/1
  Divide1/1 -> RR(2)/1
  Bus Selector/2 -> Abs1/1  "<PPR(3)>"
  Abs/1 -> R1F/1
  Abs1/1 -> R2F/1
  PPR/1 -> Bus Selector/1
  Bus Selector/1 -> Abs/1  "<PPR(1)>"
  R1F/1 -> Divide1/2
  R2F/1 -> Divide1/3
  Bus Selector/3 -> Divide1/4  "<PPR(5)>"
  [TESUB8] -> Bus Selector1/1
  Product/1 -> Divide1/1
  Math Function2/1 -> Product/1
  Bus Selector1/1 -> Product/2  "<TESUB8(8)>"

== system TEP_Final_NoScript/Reactor/Reactor Heat exchanger/Reactor Heat exchanger/Cooling water outlet temperature/TCWR Inlet temperature of cooling water °C  ==
  Add : Sum
  Bus Selector : BusSelector  OutputSignals=signal1.TESUB8(5)
  Bus Selector1 : BusSelector  OutputSignals=IDV(4)
  Constant : Constant  Value=5
  Product1 : Product
  TCWR : Outport  VectorParamsAs1DForOutWhenUnconnected=off
  wires:
  Constant/1 -> Product1/2
  Bus Selector/1 -> Add/1  "<TESUB8(5)>"
  Bus Selector1/1 -> Product1/1  "<IDV(4)>"
  [TESUB8] -> Bus Selector/1
  Product1/1 -> Add/2
  [IDV] -> Bus Selector1/1
  Add/1 -> TCWR/1

== system TEP_Final_NoScript/Reactor/Reactor Heat exchanger/Reactor Heat exchanger/Subsystem/If Action Subsystem ==
  In1 : Inport
  Action Port : ActionPort  ActionPortLabel=if(u1 > 50)
  Out1 : Outport  VectorParamsAs1DForOutWhenUnconnected=off
  wires:
  In1/1 -> Out1/1

== system TEP_Final_NoScript/Reactor/Reactor Heat exchanger/Reactor Heat exchanger/Subsystem/If Action Subsystem1 ==
  In1 : Inport
  Action Port : ActionPort  ActionPortLabel=elseif(u1 < 10)
  Out1 : Outport  VectorParamsAs1DForOutWhenUnconnected=off
  wires:
  In1/1 -> Out1/1

== system TEP_Final_NoScript/Reactor/Reactor Heat exchanger/Reactor Heat exchanger/Subsystem/If Action Subsystem2 ==
  In1 : Inport
  Action Port : ActionPort  ActionPortLabel=else
  Out1 : Outport  VectorParamsAs1DForOutWhenUnconnected=off
  wires:
  In1/1 -> Out1/1

== system TEP_Final_NoScript/Separator/Stream 9/Subsystem/Pressure drop/If Action Subsystem ==
  In1 : Inport
  Action Port : ActionPort  ActionPortLabel=if(u1 < 0)
  Out1 : Outport  VectorParamsAs1DForOutWhenUnconnected=off
  wires:
  In1/1 -> Out1/1

== system TEP_Final_NoScript/Separator/Stream 9/Subsystem/Pressure drop/If Action Subsystem1 ==
  In1 : Inport
  Action Port : ActionPort  ActionPortLabel=else
  Out1 : Outport  VectorParamsAs1DForOutWhenUnconnected=off
  wires:
  In1/1 -> Out1/1

== system TEP_Final_NoScript/Subsystem/Braatz/ 10/CONTROL 6/P Control ==
  SETPT : Inport
  GAIN : Inport  Port=2
  XMEAS : Inport  Port=3
  High Limit : Inport  Port=4
  XMV_0 : Inport  Port=5
  Action Port : ActionPort  ActionPortLabel=if(u1 == 0)
  " " : Subsystem
  ERR : Subsystem
  Subsystem : Subsystem
  XMV_NEW : Outport  VectorParamsAs1DForOutWhenUnconnected=off
  wires:
  High Limit/1 -> ERR/2(High Limit)
  GAIN/1 -> Subsystem/2(GAIN)
  " "/1(XMV) -> XMV_NEW/1
  SETPT/1 -> ERR/1(SETPT)
  Subsystem/1(DXMV) -> " "/1(DXMV)  "DXMV"
  ERR/1(ERR) -> Subsystem/1(ERR)
  XMEAS/1 -> ERR/3(XMEAS), " "/3(XMEAS)
  XMV_0/1 -> " "/2(XMV_0)

== system TEP_Final_NoScript/Subsystem1/A and C feed stream/Composition measurement mol%/Subsystem/Subsystem ==
  XST : Inport
  Constant : Constant  Value=100
  Multiport Selector : dspindex/Multiport Selector  rowsOrCols=Rows  idxCellArray={ 1,2,3,4,5,6,7,8}  idxErrMode=Clip Index
  Product{,1..7} (8 alike) : Product
  XCMPA : Outport  VectorParamsAs1DForOutWhenUnconnected=off
  XCMPB : Outport  Port=2  VectorParamsAs1DForOutWhenUnconnected=off
  XCMPC : Outport  Port=3  VectorParamsAs1DForOutWhenUnconnected=off
  XCMPD : Outport  Port=4  VectorParamsAs1DForOutWhenUnconnected=off
  "XCMPE " : Outport  Port=5  VectorParamsAs1DForOutWhenUnconnected=off
  "XCMPF " : Outport  Port=6  VectorParamsAs1DForOutWhenUnconnected=off
  XCMPG : Outport  Port=7  VectorParamsAs1DForOutWhenUnconnected=off
  "XCMPH " : Outport  Port=8  VectorParamsAs1DForOutWhenUnconnected=off
  wires:
  Multiport Selector/6 -> Product5/1
  Multiport Selector/8 -> Product7/1
  Multiport Selector/5 -> Product4/1
  Multiport Selector/7 -> Product6/1
  Multiport Selector/1 -> Product/1
  Multiport Selector/3 -> Product2/1
  Constant/1 -> Product/2, Product1/2, Product2/2, Product3/2, Product4/2, Product5/2, Product7/2, Product6/2
  Multiport Selector/4 -> Product3/1
  XST/1 -> Multiport Selector/1
  Multiport Selector/2 -> Product1/1
  Product/1 -> XCMPA/1
  Product1/1 -> XCMPB/1
  Product2/1 -> XCMPC/1
  Product3/1 -> XCMPD/1
  Product4/1 -> "XCMPE "/1
  Product5/1 -> "XCMPF "/1
  Product6/1 -> XCMPG/1
  Product7/1 -> "XCMPH "/1

== system TEP_Final_NoScript/Subsystem1/A feed stream/Composition measurement mol%/Subsystem/Subsystem ==
  XST : Inport
  Constant : Constant  Value=100
  Multiport Selector : dspindex/Multiport Selector  rowsOrCols=Rows  idxCellArray={ 1,2,3,4,5,6,7,8}  idxErrMode=Clip Index
  Product{,1..7} (8 alike) : Product
  XCMPA : Outport  VectorParamsAs1DForOutWhenUnconnected=off
  XCMPB : Outport  Port=2  VectorParamsAs1DForOutWhenUnconnected=off
  XCMPC : Outport  Port=3  VectorParamsAs1DForOutWhenUnconnected=off
  XCMPD : Outport  Port=4  VectorParamsAs1DForOutWhenUnconnected=off
  "XCMPE " : Outport  Port=5  VectorParamsAs1DForOutWhenUnconnected=off
  "XCMPF " : Outport  Port=6  VectorParamsAs1DForOutWhenUnconnected=off
  XCMPG : Outport  Port=7  VectorParamsAs1DForOutWhenUnconnected=off
  "XCMPH " : Outport  Port=8  VectorParamsAs1DForOutWhenUnconnected=off
  wires:
  Multiport Selector/6 -> Product5/1
  Multiport Selector/8 -> Product7/1
  Multiport Selector/5 -> Product4/1
  Multiport Selector/7 -> Product6/1
  Multiport Selector/1 -> Product/1
  Multiport Selector/3 -> Product2/1
  Constant/1 -> Product/2, Product1/2, Product2/2, Product3/2, Product4/2, Product5/2, Product7/2, Product6/2
  Multiport Selector/4 -> Product3/1
  XST/1 -> Multiport Selector/1
  Multiport Selector/2 -> Product1/1
  Product/1 -> XCMPA/1
  Product1/1 -> XCMPB/1
  Product2/1 -> XCMPC/1
  Product3/1 -> XCMPD/1
  Product4/1 -> "XCMPE "/1
  Product5/1 -> "XCMPF "/1
  Product6/1 -> XCMPG/1
  Product7/1 -> "XCMPH "/1

== system TEP_Final_NoScript/Subsystem1/CCin/Subsystem3/Subsystem/Subsystem2 ==
  T1 : Inport
  T0 : Inport  Port=2
  A : Constant  Value=9.069
  Add1 : Sum  Inputs=+-
  Product1 : Product
  AT : Outport
  wires:
  Add1/1 -> Product1/2
  A/1 -> Product1/1
  T0/1 -> Add1/2
  T1/1 -> Add1/1
  Product1/1 -> AT/1

== system TEP_Final_NoScript/Subsystem1/CCin/Subsystem3/Subsystem1/Subsystem ==
  T1 : Inport
  T0 : Inport  Port=2
  A : Constant  Value=9.069
  Divide : Product  Inputs=*/
  Math Function : Math  Operator=log  SignedPower=on
  Product1 : Product
  AT : Outport
  wires:
  Product1/1 -> AT/1
  A/1 -> Product1/1
  T1/1 -> Divide/1
  T0/1 -> Divide/2
  Math Function/1 -> Product1/2
  Divide/1 -> Math Function/1

== system TEP_Final_NoScript/Subsystem1/CCout/Subsystem3/Subsystem/Subsystem2 ==
  T1 : Inport
  T0 : Inport  Port=2
  A : Constant  Value=9.069
  Add1 : Sum  Inputs=+-
  Product1 : Product
  AT : Outport
  wires:
  Add1/1 -> Product1/2
  A/1 -> Product1/1
  T0/1 -> Add1/2
  T1/1 -> Add1/1
  Product1/1 -> AT/1

== system TEP_Final_NoScript/Subsystem1/CCout/Subsystem3/Subsystem1/Subsystem ==
  T1 : Inport
  T0 : Inport  Port=2
  A : Constant  Value=9.069
  Divide : Product  Inputs=*/
  Math Function : Math  Operator=log  SignedPower=on
  Product1 : Product
  AT : Outport
  wires:
  Product1/1 -> AT/1
  A/1 -> Product1/1
  T1/1 -> Divide/1
  T0/1 -> Divide/2
  Math Function/1 -> Product1/2
  Divide/1 -> Math Function/1

== system TEP_Final_NoScript/Subsystem1/D feed stream/Composition measurement mol%/Subsystem/Subsystem ==
  XST : Inport
  Constant : Constant  Value=100
  Multiport Selector : dspindex/Multiport Selector  rowsOrCols=Rows  idxCellArray={ 1,2,3,4,5,6,7,8}  idxErrMode=Clip Index
  Product{,1..7} (8 alike) : Product
  XCMPA : Outport  VectorParamsAs1DForOutWhenUnconnected=off
  XCMPB : Outport  Port=2  VectorParamsAs1DForOutWhenUnconnected=off
  XCMPC : Outport  Port=3  VectorParamsAs1DForOutWhenUnconnected=off
  XCMPD : Outport  Port=4  VectorParamsAs1DForOutWhenUnconnected=off
  "XCMPE " : Outport  Port=5  VectorParamsAs1DForOutWhenUnconnected=off
  "XCMPF " : Outport  Port=6  VectorParamsAs1DForOutWhenUnconnected=off
  XCMPG : Outport  Port=7  VectorParamsAs1DForOutWhenUnconnected=off
  "XCMPH " : Outport  Port=8  VectorParamsAs1DForOutWhenUnconnected=off
  wires:
  Multiport Selector/6 -> Product5/1
  Multiport Selector/8 -> Product7/1
  Multiport Selector/5 -> Product4/1
  Multiport Selector/7 -> Product6/1
  Multiport Selector/1 -> Product/1
  Multiport Selector/3 -> Product2/1
  Constant/1 -> Product/2, Product1/2, Product2/2, Product3/2, Product4/2, Product5/2, Product7/2, Product6/2
  Multiport Selector/4 -> Product3/1
  XST/1 -> Multiport Selector/1
  Multiport Selector/2 -> Product1/1
  Product/1 -> XCMPA/1
  Product1/1 -> XCMPB/1
  Product2/1 -> XCMPC/1
  Product3/1 -> XCMPD/1
  Product4/1 -> "XCMPE "/1
  Product5/1 -> "XCMPF "/1
  Product6/1 -> XCMPG/1
  Product7/1 -> "XCMPH "/1

== system TEP_Final_NoScript/Subsystem1/E feed stream/Composition measurement mol%/Subsystem/Subsystem ==
  XST : Inport
  Constant : Constant  Value=100
  Multiport Selector : dspindex/Multiport Selector  rowsOrCols=Rows  idxCellArray={ 1,2,3,4,5,6,7,8}  idxErrMode=Clip Index
  Product{,1..7} (8 alike) : Product
  XCMPA : Outport  VectorParamsAs1DForOutWhenUnconnected=off
  XCMPB : Outport  Port=2  VectorParamsAs1DForOutWhenUnconnected=off
  XCMPC : Outport  Port=3  VectorParamsAs1DForOutWhenUnconnected=off
  XCMPD : Outport  Port=4  VectorParamsAs1DForOutWhenUnconnected=off
  "XCMPE " : Outport  Port=5  VectorParamsAs1DForOutWhenUnconnected=off
  "XCMPF " : Outport  Port=6  VectorParamsAs1DForOutWhenUnconnected=off
  XCMPG : Outport  Port=7  VectorParamsAs1DForOutWhenUnconnected=off
  "XCMPH " : Outport  Port=8  VectorParamsAs1DForOutWhenUnconnected=off
  wires:
  Multiport Selector/6 -> Product5/1
  Multiport Selector/8 -> Product7/1
  Multiport Selector/5 -> Product4/1
  Multiport Selector/7 -> Product6/1
  Multiport Selector/1 -> Product/1
  Multiport Selector/3 -> Product2/1
  Constant/1 -> Product/2, Product1/2, Product2/2, Product3/2, Product4/2, Product5/2, Product7/2, Product6/2
  Multiport Selector/4 -> Product3/1
  XST/1 -> Multiport Selector/1
  Multiport Selector/2 -> Product1/1
  Product/1 -> XCMPA/1
  Product1/1 -> XCMPB/1
  Product2/1 -> XCMPC/1
  Product3/1 -> XCMPD/1
  Product4/1 -> "XCMPE "/1
  Product5/1 -> "XCMPF "/1
  Product6/1 -> XCMPG/1
  Product7/1 -> "XCMPH "/1

== system TEP_Final_NoScript/Subsystem1/Product stream/Composition measurement mol%/Subsystem/Subsystem ==
  XST : Inport
  Constant : Constant  Value=100
  Multiport Selector : dspindex/Multiport Selector  rowsOrCols=Rows  idxCellArray={ 1,2,3}  idxErrMode=Clip Index
  Product : Product
  Product1 : Product
  Product2 : Product
  XCMPA : Outport  VectorParamsAs1DForOutWhenUnconnected=off
  XCMPB : Outport  Port=2  VectorParamsAs1DForOutWhenUnconnected=off
  XCMPC : Outport  Port=3  VectorParamsAs1DForOutWhenUnconnected=off
  wires:
  Multiport Selector/1 -> Product/1
  Multiport Selector/3 -> Product2/1
  Constant/1 -> Product2/2, Product/2, Product1/2
  XST/1 -> Multiport Selector/1
  Multiport Selector/2 -> Product1/1
  Product/1 -> XCMPA/1
  Product1/1 -> XCMPB/1
  Product2/1 -> XCMPC/1

== system TEP_Final_NoScript/Subsystem1/Product stream/Composition measurement mol%/Subsystem1/Subsystem ==
  XST : Inport
  Constant : Constant  Value=100
  Multiport Selector : dspindex/Multiport Selector  rowsOrCols=Rows  idxCellArray={4,5,6,7,8}  idxErrMode=Clip Index
  "XCMPD " : Product
  XCMPE : Product
  XCMPF : Product
  "XCMPG " : Product
  XCMPH : Product
  XCMPD : Outport  VectorParamsAs1DForOutWhenUnconnected=off
  "XCMPE " : Outport  Port=2  VectorParamsAs1DForOutWhenUnconnected=off
  "XCMPF " : Outport  Port=3  VectorParamsAs1DForOutWhenUnconnected=off
  XCMPG : Outport  Port=4  VectorParamsAs1DForOutWhenUnconnected=off
  "XCMPH " : Outport  Port=5  VectorParamsAs1DForOutWhenUnconnected=off
  wires:
  Constant/1 -> XCMPE/2, "XCMPG "/2, XCMPH/2, XCMPF/2, "XCMPD "/2
  Multiport Selector/1 -> "XCMPD "/1
  "XCMPD "/1 -> XCMPD/1  "XCMPD"
  Multiport Selector/5 -> XCMPH/1
  XCMPF/1 -> "XCMPF "/1  "XCMPF"
  XST/1 -> Multiport Selector/1
  Multiport Selector/4 -> "XCMPG "/1
  Multiport Selector/2 -> XCMPE/1
  Multiport Selector/3 -> XCMPF/1
  XCMPE/1 -> "XCMPE "/1  "XCMPE"
  XCMPH/1 -> "XCMPH "/1  "XCMPH"
  "XCMPG "/1 -> XCMPG/1  "XCMPG"

== system TEP_Final_NoScript/Subsystem1/RCin/Subsystem3/Subsystem/Subsystem2 ==
  T1 : Inport
  T0 : Inport  Port=2
  A : Constant  Value=9.069
  Add1 : Sum  Inputs=+-
  Product1 : Product
  AT : Outport
  wires:
  Add1/1 -> Product1/2
  A/1 -> Product1/1
  T0/1 -> Add1/2
  T1/1 -> Add1/1
  Product1/1 -> AT/1

== system TEP_Final_NoScript/Subsystem1/RCin/Subsystem3/Subsystem1/Subsystem ==
  T1 : Inport
  T0 : Inport  Port=2
  A : Constant  Value=9.069
  Divide : Product  Inputs=*/
  Math Function : Math  Operator=log  SignedPower=on
  Product1 : Product
  AT : Outport
  wires:
  Product1/1 -> AT/1
  A/1 -> Product1/1
  T1/1 -> Divide/1
  T0/1 -> Divide/2
  Math Function/1 -> Product1/2
  Divide/1 -> Math Function/1
